simulink model "gm_MASH_HDL"  (R2013b)
settings: Solver=FixedStepDiscrete  SolverMode=SingleTasking  StartTime=0.0  StopTime=N/Fs  RelTol=1e-3
undefined symbols (not defined in the file or in its folder): nLev
settings Model: Creator=o_cotte  LastModifiedBy=o_cotte
settings OptimizationCC: BlockReduction=off  BooleanDataType=off  ConditionallyExecuteInputs=off
settings DebuggingCC: SaveWithParameterizedLinksMsg=none  SignalResolutionControl=TryResolveAllWithWarning  SolverPrmCheckMsg=none  MultiTaskDSMMsg=warning  MultiTaskCondExecSysMsg=none
settings HardwareCC: TargetUnknown=on
settings RTWCC: IncludeERTFirstTime=on

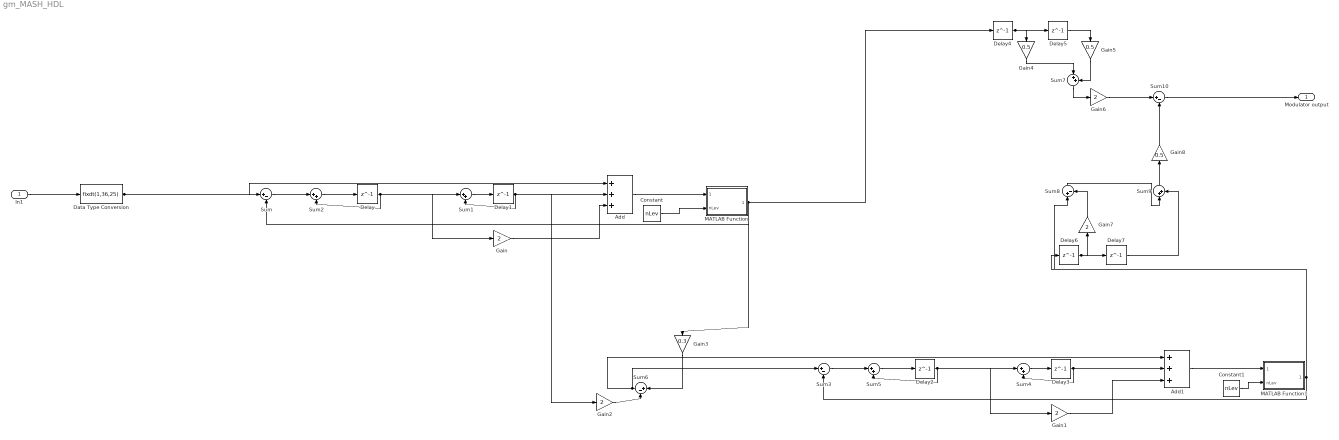
== system gm_MASH_HDL ==
  In1 : Inport
  Add : Sum  Inputs=+++  OutDataTypeStr=Inherit: Same as accumulator  LockScale=on
  Add1 : Sum  Inputs=+++  OutDataTypeStr=Inherit: Same as accumulator  LockScale=on
  Constant : Constant  Value=nLev
  Constant1 : Constant  Value=nLev
  Data Type Conversion : DataTypeConversion  OutDataTypeStr=fixdt(1,36,25)  LockScale=on
  Delay{,1..7} (8 alike) : Delay  DelayLength=1  InitialCondition=0
  Gain : Gain  Gain=2  OutDataTypeStr=Inherit: Same as input  LockScale=on
  Gain1 : Gain  Gain=2  OutDataTypeStr=Inherit: Same as input  LockScale=on
  Gain2 : Gain  Gain=2  OutDataTypeStr=fixdt(1,34,23)
  Gain3 : Gain  Gain=0.3  OutDataTypeStr=Inherit: Same as input  LockScale=on
  Gain4 : Gain  Gain=0.5  OutDataTypeStr=Inherit: Same as input  ParamDataTypeStr=Inherit: Same as input  LockScale=on
  Gain5 : Gain  Gain=0.5  OutDataTypeStr=Inherit: Same as input  ParamDataTypeStr=Inherit: Same as input  LockScale=on
  Gain6 : Gain  Gain=2  OutDataTypeStr=Inherit: Same as input  LockScale=on
  Gain7 : Gain  Gain=2  OutDataTypeStr=fixdt(1,34,23)
  Gain8 : Gain  Gain=0.5  OutDataTypeStr=Inherit: Same as input  ParamDataTypeStr=Inherit: Same as input  LockScale=on
  MATLAB Function : Subsystem
  MATLAB Function1 : Subsystem
  Sum{,3,6,8,10} (5 alike) : Sum  Inputs=|+-  OutDataTypeStr=Inherit: Same as accumulator  LockScale=on
  Sum{1..2,4..5,7,9} (6 alike) : Sum  Inputs=|++  OutDataTypeStr=Inherit: Same as accumulator  LockScale=on
  Modulator output : Outport
  wires:
  In1/1 -> Data Type Conversion/1
  Add/1 -> MATLAB Function/1(quant_in)
  Add1/1 -> MATLAB Function1/1(quant_in)
  Constant/1 -> MATLAB Function/2(nLev)
  Constant1/1 -> MATLAB Function1/2(nLev)
  Data Type Conversion/1 -> Sum/1, Add/1
  Delay/1 -> Sum2/2, Sum1/1, Gain/1
  Delay1/1 -> Sum1/2, Gain2/1, Add/2
  Delay2/1 -> Sum5/2, Sum4/1, Gain1/1
  Delay3/1 -> Sum4/2, Add1/2
  Delay4/1 -> Gain4/1, Delay5/1
  Delay5/1 -> Gain5/1
  Delay6/1 -> Gain7/1, Delay7/1
  Delay7/1 -> Sum9/2
  Gain/1 -> Add/3
  Gain1/1 -> Add1/3
  Gain2/1 -> Sum6/2
  Gain3/1 -> Sum6/1
  Gain4/1 -> Sum7/1
  Gain5/1 -> Sum7/2
  Gain6/1 -> Sum10/1
  Gain7/1 -> Sum8/2
  Gain8/1 -> Sum10/2
  MATLAB Function/1(quant_out) -> Sum/2, Gain3/1, Delay4/1
  MATLAB Function1/1(quant_out) -> Sum8/1, Sum3/2, Delay6/1
  Sum/1 -> Sum2/1
  Sum1/1 -> Delay1/1
  Sum10/1 -> Modulator output/1
  Sum2/1 -> Delay/1
  Sum3/1 -> Sum5/1
  Sum4/1 -> Delay3/1
  Sum5/1 -> Delay2/1
  Sum6/1 -> Sum3/1, Add1/1
  Sum7/1 -> Gain6/1
  Sum8/1 -> Sum9/1
  Sum9/1 -> Gain8/1

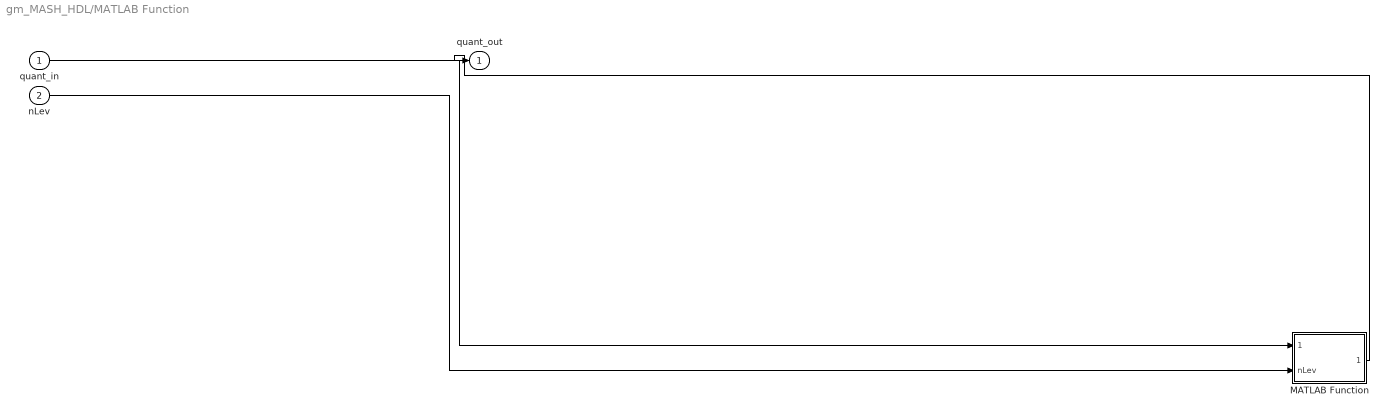
== system gm_MASH_HDL/MATLAB Function ==
  quant_in : Inport
  nLev : Inport  Port=2
  MATLAB Function : MATLAB Function  TreatAsAtomicUnit=on
  quant_out : Outport
  wires:
  quant_in/1 -> MATLAB Function/1(quant_in)
  nLev/1 -> MATLAB Function/2(nLev)
  MATLAB Function/1(quant_out) -> quant_out/1

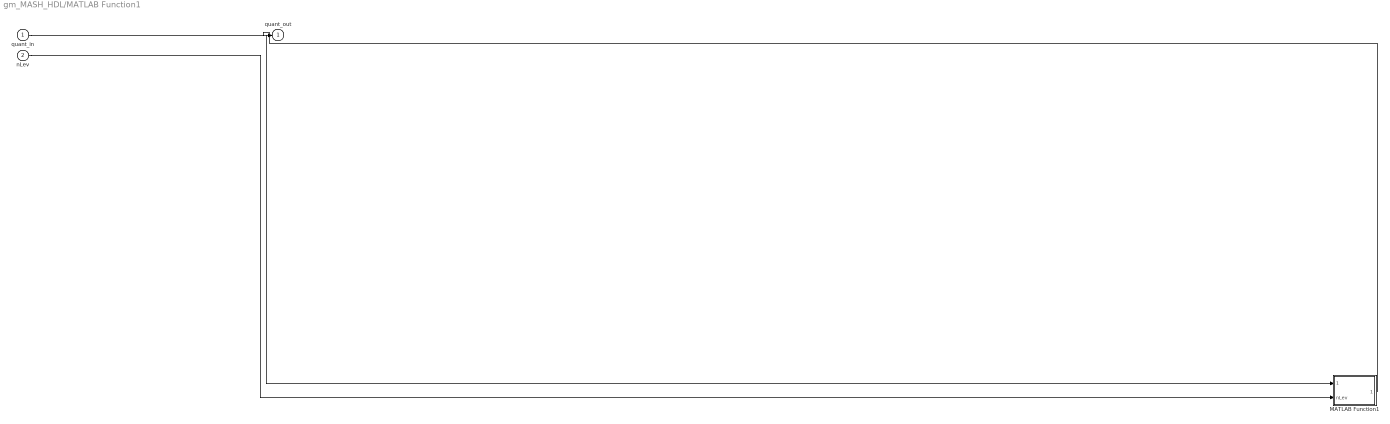
== system gm_MASH_HDL/MATLAB Function1 ==
  quant_in : Inport
  nLev : Inport  Port=2
  MATLAB Function1 : MATLAB Function  TreatAsAtomicUnit=on
  quant_out : Outport
  wires:
  quant_in/1 -> MATLAB Function1/1(quant_in)
  nLev/1 -> MATLAB Function1/2(nLev)
  MATLAB Function1/1(quant_out) -> quant_out/1

== matlab function gm_MASH_HDL/MATLAB Function1/MATLAB Function1 ==
  data: quant_in input; quant_out output; nLev input
function quant_out = fcn(quant_in,nLev)
%#codegen
% st=fi(nLev-2,1,34,22);
% quant_out=fi(0,1,34,22);
% if quant_in < -st
%     quant_out = fi(-nLev+1,1,34,22);
%     %     return;
% elseif quant_in >= st
%     quant_out = fi(nLev-1,1,34,22);
%     %     return;
% else
%     for n=1:nLev-2
%         k=fi(n,1,34,22);
%         if quant_in >= -nLev + 2*k && quant_in < -nLev + 2*(k+1)
%             quant_out = fi(2*k-1-nLev,1,34,22);
%         end
%     end
% end

if quant_in < 0
    quant_out = fi(-1,1,36,25);
    %y = -1;
else
    quant_out = fi(1,1,36,25);
    %y = 1;
end

== matlab function gm_MASH_HDL/MATLAB Function/MATLAB Function ==
  data: quant_in input; quant_out output; nLev input
function quant_out = fcn(quant_in,nLev)
%#codegen
% st=fi(nLev-2,1,34,22);
% quant_out=fi(0,1,34,22);
% if quant_in < -st
%     quant_out = fi(-nLev+1,1,34,22);
%     %     return;
% elseif quant_in >= st
%     quant_out = fi(nLev-1,1,34,22);
%     %     return;
% else
%     for n=1:nLev-2
%         k=fi(n,1,34,22);
%         if quant_in >= -nLev + 2*k && quant_in < -nLev + 2*(k+1)
%             quant_out = fi(2*k-1-nLev,1,34,22);
%         end
%     end
% end

if quant_in < 0
    quant_out = fi(-1,1,36,25);
    %y = -1;
else
    quant_out = fi(1,1,36,25);
    %y = 1;
end
